simulink model "Quat_Test"  (Simulink 7.5)
settings: Solver=ode45  StartTime=0.0  StopTime=10.0  RelTol=1e-3
values from neighbouring files (symbols this model uses):
  apSampleTime = 0.01    [demoz2SlugsV5.m]
  QUAT_0 = DCM2Quat( R0 )    [demoz2SlugsV5.m]
undefined symbols (not defined in the file or in its folder): DiscIntNeverNeededParam
libraries: aerolibutil x2
settings Model: Creator=Robert  LastModifiedBy=Robert

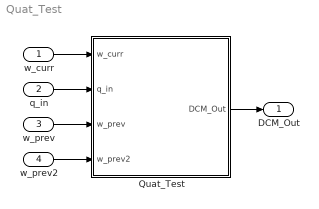
== system Quat_Test ==
  w_curr : Inport  DataType=single  OutDataType=fixdt(1, 16)  OutScaling=2^0  OutDataTypeStr=single
  q_in : Inport  Port=2  DataType=single  OutDataType=fixdt(1, 16)  OutScaling=2^0  OutDataTypeStr=single
  w_prev : Inport  Port=3  DataType=single  OutDataType=fixdt(1, 16)  OutScaling=2^0  OutDataTypeStr=single
  w_prev2 : Inport  Port=4  DataType=single  OutDataType=fixdt(1, 16)  OutScaling=2^0  OutDataTypeStr=single
  Quat_Test : Subsystem
  DCM_Out : Outport  OutDataType=fixdt(1, 16)  OutScaling=2^0
  wires:
  w_curr/1 -> Quat_Test/1(w_curr)
  q_in/1 -> Quat_Test/2(q_in)
  w_prev/1 -> Quat_Test/3(w_prev)
  Quat_Test/1(DCM_Out) -> DCM_Out/1
  w_prev2/1 -> Quat_Test/4(w_prev2)

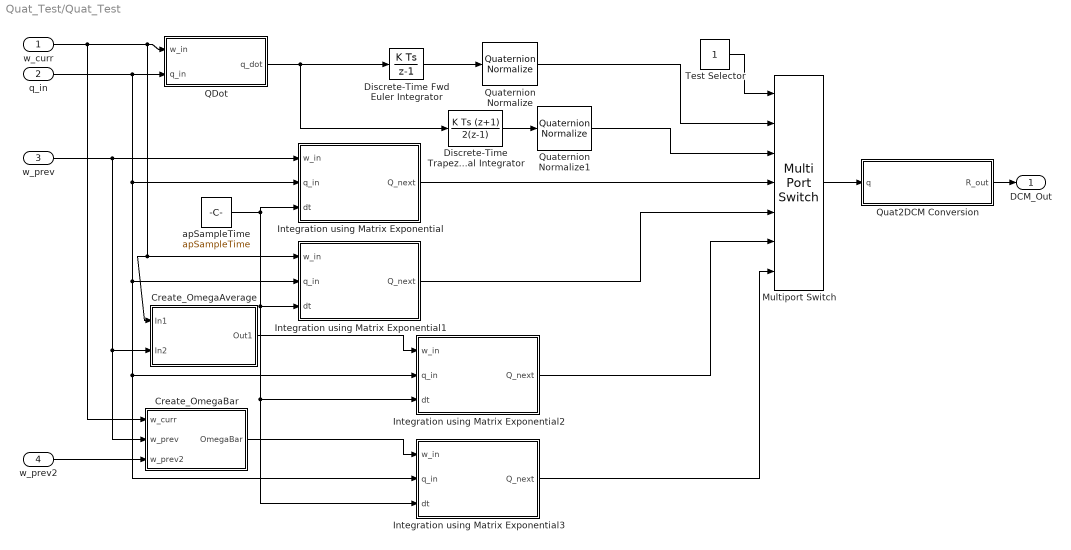
== system Quat_Test/Quat_Test ==
  w_curr : Inport  DataType=single  OutDataType=fixdt(1, 16)  OutScaling=2^0  OutDataTypeStr=single
  q_in : Inport  Port=2  DataType=single  OutDataType=fixdt(1, 16)  OutScaling=2^0  OutDataTypeStr=single
  w_prev : Inport  Port=3  DataType=single  OutDataType=fixdt(1, 16)  OutScaling=2^0  OutDataTypeStr=single
  w_prev2 : Inport  Port=4  DataType=single  OutDataType=fixdt(1, 16)  OutScaling=2^0  OutDataTypeStr=single
  Create_OmegaAverage : Subsystem
  Create_OmegaBar : Subsystem
  Discrete-Time Fwd Euler Integrator : DiscreteIntegrator  InitialCondition=QUAT_0  SampleTime=apSampleTime  OutDataTypeMode=single  OutDataType=fixdt(1, 16)  OutScaling=2^0  OutDataTypeStr=single  ICPrevOutput=DiscIntNeverNeededParam  ICPrevScaledInput=DiscIntNeverNeededParam
  Discrete-Time Trapezoidal Integrator : DiscreteIntegrator  IntegratorMethod=Integration: Trapezoidal  InitialCondition=QUAT_0  SampleTime=apSampleTime  OutDataTypeMode=single  OutDataType=fixdt(1, 16)  OutScaling=2^0  OutDataTypeStr=single  ICPrevOutput=DiscIntNeverNeededParam  ICPrevScaledInput=DiscIntNeverNeededParam
  Integration using Matrix Exponential : Stateflow chart  TreatAsAtomicUnit=on
  Integration using Matrix Exponential1 : Stateflow chart  TreatAsAtomicUnit=on
  Integration using Matrix Exponential2 : Stateflow chart  TreatAsAtomicUnit=on
  Integration using Matrix Exponential3 : Stateflow chart  TreatAsAtomicUnit=on
  Multiport Switch : MultiPortSwitch  Inputs=6  zeroidx=off  OutDataType=fixdt(1, 16)  OutScaling=2^0
  QDot : Stateflow chart  TreatAsAtomicUnit=on
  Quat2DCM Conversion : Stateflow chart  TreatAsAtomicUnit=on
  Quaternion Normalize : aerolibutil/Quaternion Normalize  SystemSampleTime=-1
  Quaternion Normalize1 : aerolibutil/Quaternion Normalize  SystemSampleTime=-1
  Test Selector : Constant  OutDataType=fixdt(1, 16)  OutScaling=2^0
  apSampleTime : Constant  Value=apSampleTime  OutDataTypeMode=single  OutDataType=fixdt(1, 16)  OutScaling=2^0  OutDataTypeStr=single
  DCM_Out : Outport  OutDataType=fixdt(1, 16)  OutScaling=2^0
  wires:
  w_curr/1 -> QDot/1(w_in), Integration using Matrix Exponential1/1(w_in), Create_OmegaAverage/1(In1), Create_OmegaBar/1(w_curr)
  q_in/1 -> QDot/2(q_in), Integration using Matrix Exponential/2(q_in), Integration using Matrix Exponential1/2(q_in), Integration using Matrix Exponential3/2(q_in), Integration using Matrix Exponential2/2(q_in)
  QDot/1(q_dot) -> Discrete-Time Fwd Euler Integrator/1, Discrete-Time Trapezoidal Integrator/1
  Test Selector/1 -> Multiport Switch/1
  Discrete-Time Fwd Euler Integrator/1 -> Quaternion Normalize/1
  Discrete-Time Trapezoidal Integrator/1 -> Quaternion Normalize1/1
  Multiport Switch/1 -> Quat2DCM Conversion/1(q)
  Quat2DCM Conversion/1(R_out) -> DCM_Out/1
  Integration using Matrix Exponential/1(Q_next) -> Multiport Switch/4
  Integration using Matrix Exponential1/1(Q_next) -> Multiport Switch/5
  Integration using Matrix Exponential2/1(Q_next) -> Multiport Switch/6
  Integration using Matrix Exponential3/1(Q_next) -> Multiport Switch/7
  w_prev/1 -> Integration using Matrix Exponential/1(w_in), Create_OmegaAverage/2(In2), Create_OmegaBar/2(w_prev)
  apSampleTime/1 -> Integration using Matrix Exponential/3(dt), Integration using Matrix Exponential1/3(dt), Integration using Matrix Exponential2/3(dt), Integration using Matrix Exponential3/3(dt)
  Create_OmegaAverage/1(Out1) -> Integration using Matrix Exponential2/1(w_in)
  Create_OmegaBar/1(OmegaBar) -> Integration using Matrix Exponential3/1(w_in)
  w_prev2/1 -> Create_OmegaBar/3(w_prev2)
  Quaternion Normalize/1 -> Multiport Switch/2
  Quaternion Normalize1/1 -> Multiport Switch/3

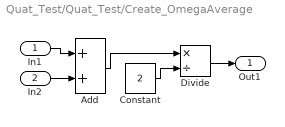
== system Quat_Test/Quat_Test/Create_OmegaAverage ==
  In1 : Inport
  In2 : Inport  Port=2
  Add : Sum  OutDataType=fixdt(1, 16)  OutScaling=2^-10
  Constant : Constant  Value=2  OutDataTypeMode=single  OutDataType=fixdt(1, 16)  OutScaling=2^0  OutDataTypeStr=single
  Divide : Product  Inputs=*/  OutDataType=fixdt(1, 16)  OutScaling=2^-10
  Out1 : Outport
  wires:
  Constant/1 -> Divide/2
  Add/1 -> Divide/1
  In1/1 -> Add/1
  In2/1 -> Add/2
  Divide/1 -> Out1/1

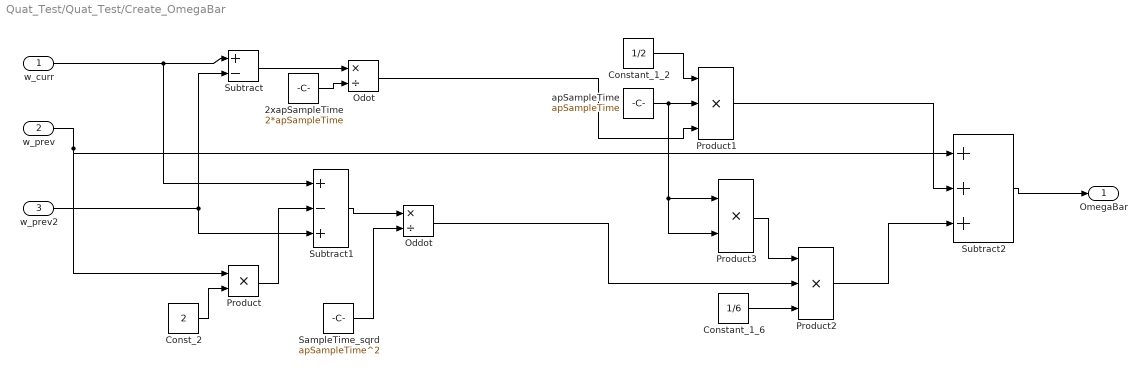
== system Quat_Test/Quat_Test/Create_OmegaBar ==
  w_curr : Inport
  w_prev : Inport  Port=2
  w_prev2 : Inport  Port=3
  2xapSampleTime : Constant  Value=2*apSampleTime  OutDataTypeMode=single  OutDataType=fixdt(1, 16)  OutScaling=2^0  OutDataTypeStr=single
  Const_2 : Constant  Value=2  OutDataTypeMode=single  OutDataType=fixdt(1, 16)  OutScaling=2^0  OutDataTypeStr=single
  Constant_1_2 : Constant  Value=1/2  OutDataTypeMode=single  OutDataType=fixdt(1, 16)  OutScaling=2^0  OutDataTypeStr=single
  Constant_1_6 : Constant  Value=1/6  OutDataTypeMode=single  OutDataType=fixdt(1, 16)  OutScaling=2^0  OutDataTypeStr=single
  Oddot : Product  Inputs=*/  OutDataType=fixdt(1, 16)  OutScaling=2^-10
  Odot : Product  Inputs=*/  OutDataType=fixdt(1, 16)  OutScaling=2^-10
  Product : Product  OutDataType=fixdt(1, 16)  OutScaling=2^0  RndMeth=Zero
  Product1 : Product  Inputs=3  OutDataType=fixdt(1, 16)  OutScaling=2^0  RndMeth=Zero
  Product2 : Product  Inputs=3  OutDataType=fixdt(1, 16)  OutScaling=2^0  RndMeth=Zero
  Product3 : Product  OutDataTypeMode=single  OutDataType=fixdt(1, 16)  OutScaling=2^0  OutDataTypeStr=single  SampleTime=apSampleTime  RndMeth=Zero
  SampleTime_sqrd : Constant  Value=apSampleTime^2  OutDataTypeMode=single  OutDataType=fixdt(1, 16)  OutScaling=2^0  OutDataTypeStr=single
  Subtract : Sum  Inputs=+-  OutDataType=fixdt(1, 16)  OutScaling=2^-10
  Subtract1 : Sum  Inputs=+-+  OutDataType=fixdt(1, 16)  OutScaling=2^-10
  Subtract2 : Sum  Inputs=+++  OutDataTypeMode=single  OutDataType=fixdt(1, 16)  OutScaling=2^-10  OutDataTypeStr=single
  apSampleTime : Constant  Value=apSampleTime  OutDataTypeMode=single  OutDataType=fixdt(1, 16)  OutScaling=2^0  OutDataTypeStr=single
  OmegaBar : Outport
  wires:
  w_prev/1 -> Product/1, Subtract2/1
  w_curr/1 -> Subtract/1, Subtract1/1
  w_prev2/1 -> Subtract/2, Subtract1/3
  Subtract/1 -> Odot/1
  2xapSampleTime/1 -> Odot/2
  SampleTime_sqrd/1 -> Oddot/2
  Subtract1/1 -> Oddot/1
  Const_2/1 -> Product/2
  Product/1 -> Subtract1/2
  Subtract2/1 -> OmegaBar/1
  Constant_1_2/1 -> Product1/1
  apSampleTime/1 -> Product1/2, Product3/1, Product3/2
  Odot/1 -> Product1/3
  Product1/1 -> Subtract2/2
  Constant_1_6/1 -> Product2/3
  Product3/1 -> Product2/1
  Oddot/1 -> Product2/2
  Product2/1 -> Subtract2/3

== matlab function Quat_Test/Quat2DCM Conversion ==
  data: q input double; R_out output double
function R_out = Quat2DCM( q )
%#eml
%QUAT2DCM Function converts quaternion into direction cosine matrix
%   q = input quaternion (q(1-4)); can be row vector or column vector
%   R_out = output DCM, 3x3 matrix
%   q(1) is the scalar part, q(2-4) form the vector part.
%   Using conversion formula from Ch.7, Sect.7 (pg. 168) of 
%   J. Kuipers "Quaternions and Rotation Sequences."

R_out = single(zeros( 3, 3 )); % memory alloc

R_out = [ 2*q(1)^2 - 1 + 2*q(2)^2      2*q(2)*q(3) + 2*q(1)*q(4)   2*q(2)*q(4) - 2*q(1)*q(3); ...
        2*q(2)*q(3) - 2*q(1)*q(4)      2*q(1)^2 - 1 + 2*q(3)^2     2*q(3)*q(4) + 2*q(1)*q(2); ...
        2*q(2)*q(4) + 2*q(1)*q(3)      2*q(3)*q(4) - 2*q(1)*q(2)   2*q(1)^2 - 1 + 2*q(4)^2 ];
end

== matlab function Quat_Test/QDot ==
  data: w_in input double; q_dot output double; q_in input double
function q_dot   = QDot( w_in, q_in )
%#eml
%QDOT Function calculates the change in the rotation quaternion, q_dot
%   INPUTS
%   w_in - the body-fixed angular velocities, 3x1 pqr
%   q_in - the initial 4x1 quaternion, where q_in(1) scalar, q_in(2:4) vector
%   RETVAL
%   q_dot - the 4x1 vector of changes in the rotation quaternion
%   Formulation from P. Zipfel "Modeling and Simulation of Aerospace
%   Vehicle Dynamics", Eq. 4.77
p = w_in(1);
q = w_in(2);
r = w_in(3);
q_dot = single(zeros( 4, 1 ));
q_dot = (1/2) * [ 0 -p -q -r; p 0 r -q; q -r 0 p; r q -p 0 ] * q_in;

end

== matlab function Quat_Test/Integration using Matrix Exponential ==
  data: w_in input double; Q_next output double; q_in input double; dt input double
function Q_next = QMexp( w_in, q_in, dt )
%#eml
% Q_NEXT Function performs integration of the rotation quaternion
%   using the matrix exponential.
%
%   PARAMETERS
%   w_in - pqr angular velocities in body-fixed frame
%   q_in - 4x1 vector of the current attitude quaternion, q_n
%   dt - time step between samples
%   RETVAL
%   Q_next - 4x1 vector representing the value of the next quaternion 

% Formula from Eq. 17-18 of J. Wertz, 
% 'Spacecraft Attitude Determination and Control', 1978
I4 = single(eye( 4 ));
p = w_in(1);
q = w_in(2);
r = w_in(3);
Omega = [ 0 -p -q -r; p 0 r -q; q -r 0 p; r q -p 0 ];
wn = sqrt( p^2 + q^2 + r^2 );

% Closed-form integration
if( wn ~= 0 )
    Q_next = ( cos( ( wn * dt )/ 2 ) * I4 + ...
        (1/wn) * sin( wn * dt / 2 ) * Omega ) * q_in;
else
    Q_next = q_in; % (wn == 0) --> no change in q_in
end % if

end

== matlab function Quat_Test/Integration using Matrix Exponential1 ==
  data: w_in input double; Q_next output double; q_in input double; dt input double
function Q_next = QMexp( w_in, q_in, dt )
%#eml
% Q_NEXT Function performs integration of the rotation quaternion
%   using the matrix exponential.
%
%   PARAMETERS
%   w_in - pqr angular velocities in body-fixed frame
%   q_in - 4x1 vector of the current attitude quaternion, q_n
%   dt - time step between samples
%   RETVAL
%   Q_next - 4x1 vector representing the value of the next quaternion 

% Formula from Eq. 17-18 of J. Wertz, 
% 'Spacecraft Attitude Determination and Control', 1978
I4 = single(eye( 4 ));
p = w_in(1);
q = w_in(2);
r = w_in(3);
Omega = [ 0 -p -q -r; p 0 r -q; q -r 0 p; r q -p 0 ];
wn = sqrt( p^2 + q^2 + r^2 );

% Closed-form integration
if( wn ~= 0 )
    Q_next = ( cos( ( wn * dt )/ 2 ) * I4 + ...
        (1/wn) * sin( wn * dt / 2 ) * Omega ) * q_in;
else
    Q_next = q_in; % (wn == 0) --> no change in q_in
end % if

end

== matlab function Quat_Test/Integration using Matrix Exponential2 ==
  data: w_in input double; Q_next output double; q_in input double; dt input double
function Q_next = QMexp( w_in, q_in, dt )
%#eml
% Q_NEXT Function performs integration of the rotation quaternion
%   using the matrix exponential.
%
%   PARAMETERS
%   w_in - pqr angular velocities in body-fixed frame
%   q_in - 4x1 vector of the current attitude quaternion, q_n
%   dt - time step between samples
%   RETVAL
%   Q_next - 4x1 vector representing the value of the next quaternion 

% Formula from Eq. 17-18 of J. Wertz, 
% 'Spacecraft Attitude Determination and Control', 1978
I4 = single(eye( 4 ));
p = w_in(1);
q = w_in(2);
r = w_in(3);
Omega = [ 0 -p -q -r; p 0 r -q; q -r 0 p; r q -p 0 ];
wn = sqrt( p^2 + q^2 + r^2 );

% Closed-form integration
if( wn ~= 0 )
    Q_next = ( cos( ( wn * dt )/ 2 ) * I4 + ...
        (1/wn) * sin( wn * dt / 2 ) * Omega ) * q_in;
else
    Q_next = q_in; % (wn == 0) --> no change in q_in
end % if

end

== matlab function Quat_Test/Integration using Matrix Exponential3 ==
  data: w_in input double; Q_next output double; q_in input double; dt input double
function Q_next = QMexp( w_in, q_in, dt )
%#eml
% Q_NEXT Function performs integration of the rotation quaternion
%   using the matrix exponential.
%
%   PARAMETERS
%   w_in - pqr angular velocities in body-fixed frame
%   q_in - 4x1 vector of the current attitude quaternion, q_n
%   dt - time step between samples
%   RETVAL
%   Q_next - 4x1 vector representing the value of the next quaternion 

% Formula from Eq. 17-18 of J. Wertz, 
% 'Spacecraft Attitude Determination and Control', 1978
I4 = single(eye( 4 ));
p = w_in(1);
q = w_in(2);
r = w_in(3);
Omega = [ 0 -p -q -r; p 0 r -q; q -r 0 p; r q -p 0 ];
wn = sqrt( p^2 + q^2 + r^2 );

% Closed-form integration
if( wn ~= 0 )
    Q_next = ( cos( ( wn * dt )/ 2 ) * I4 + ...
        (1/wn) * sin( wn * dt / 2 ) * Omega ) * q_in;
else
    Q_next = q_in; % (wn == 0) --> no change in q_in
end % if

end
